simulink model "model1"  (R2019a)
settings: Solver=ode4  StartTime=0.0  StopTime=10.0  FixedStep=1E-3  RelTol=1e-3
values from neighbouring files (symbols this model uses):
  Kd = [3.0237 2.7708 7.5699 12.4043 5.742]    [code.m]    (also in matlab.mat)
  Ki = [1.5240 2.9039 1.9780 1.6885 2.8586]    [code.m]    (also in matlab.mat = [1.524 2.9039 1.978 1.6885 2.8586])
  Kp = [128.5204 102.3185 111.2328 109.4094 98.049]    [code.m]    (also in matlab.mat)
  Sce = Kd./(Kp*e_max)    [code.m]    (also in matlab.mat = [0.00235270042733 0.00270801467965 0.00680545666386 0.011337)
  Se = 1/e_max    (= 0.1)    [code.m]    (also in matlab.mat)
  Sie = Ki./(Kp*e_max)    [code.m]    (also in matlab.mat = [0.00118580396575 0.00283809868206 0.00177825245791 0.001543)
  Sout = e_max.*Kp    [code.m]    (also in matlab.mat = [1285.204 1023.185 1112.328 1094.094 980.49])
libraries: Fuzzy_Type2_Lib x5, simulink x5
settings Model: Creator=LENOVO  LastModifiedBy=LENOVO
settings DebuggingCC: UnderSpecifiedDimensionMsg=warning

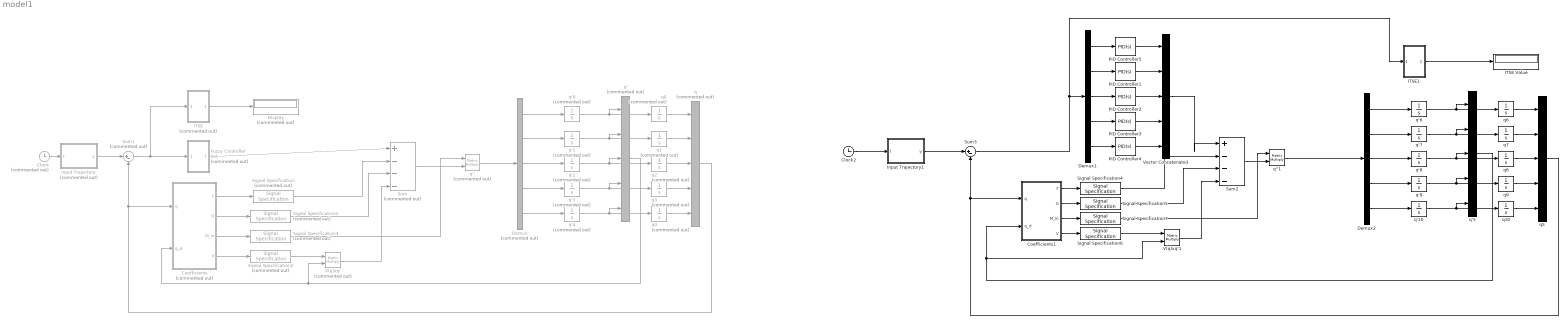
== system model1 ==
  Clock : Clock  Commented=on
  Clock2 : Clock
  Coefficients : MATLAB Function  Commented=on  TreatAsAtomicUnit=on
  Coefficients1 : MATLAB Function  TreatAsAtomicUnit=on
  Demux : Demux  Commented=on  Outputs=5
  Demux1 : Demux  Outputs=5
  Demux2 : Demux  Outputs=5
  Display : Display  Commented=on
  Fuzzy Controller Set : Subsystem  Commented=on
  ITSE : Subsystem  Commented=on
  ITSE Value : Display
  ITSE1 : Subsystem
  Input Trajectory : MATLAB Function  Commented=on  TreatAsAtomicUnit=on
  Input Trajectory1 : MATLAB Function  TreatAsAtomicUnit=on
  PID Controller1 : simulink/Continuous/PID Controller  Controller=PID  Form=Parallel  TimeDomain=Continuous-time  SampleTime=-1  IntegratorMethod=Forward Euler  FilterMethod=Forward Euler  ControllerParametersSource=internal  P=Kp(2)  I=Ki(2)  D=Kd(2)  UseFilter=on  N=100  TunerSelectOption=Transfer Function Based (PID Tuner App)  InitialConditionSource=internal  InitialConditionForIntegrator=0  InitialConditionForFilter=0  DifferentiatorICPrevScaledInput=0  ExternalReset=none  TrackingMode=off  Kt=1  LimitOutput=off  UpperSaturationLimit=inf  LowerSaturationLimit=-inf  LinearizeAsGain=on  AntiWindupMode=none  Kb=1  POutMin=[]  POutMax=[]  IOutMin=[]  IOutMax=[]  DOutMin=[]  DOutMax=[]  NOutMin=[]  NOutMax=[]  SumOutMin=[]  SumOutMax=[]  SaturationOutMin=[]  SaturationOutMax=[]  PParamMin=[]  PParamMax=[]  IParamMin=[]  IParamMax=[]  DParamMin=[]  DParamMax=[]  NParamMin=[]  NParamMax=[]  KbParamMin=[]  KbParamMax=[]  KtParamMin=[]  KtParamMax=[]  KbOutMin=[]  KbOutMax=[]  KtOutMin=[]  KtOutMax=[]  IntegratorOutMin=[]  IntegratorOutMax=[]  FilterOutMin=[]  FilterOutMax=[]  SumI1OutMin=[]  SumI1OutMax=[]  SumI2OutMin=[]  SumI2OutMax=[]  SumI3OutMin=[]  SumI3OutMax=[]  SumI4OutMin=[]  SumI4OutMax=[]  SumDOutMin=[]  SumDOutMax=[]  DifferentiatorOutMin=[]  DifferentiatorOutMax=[]  FilterDiffOutCoefMin=[]  FilterDiffOutCoefMax=[]  ReciprocalOutMin=[]  ReciprocalOutMax=[]  SumDenOutMin=[]  SumDenOutMax=[]  SumNumOutMin=[]  SumNumOutMax=[]  DivideOutMin=[]  DivideOutMax=[]  IntegratorContinuousStateAttributes=''  IntegratorStateMustResolveToSignalObject=off  IntegratorRTWStateStorageClass=Auto  FilterContinuousStateAttributes=''  FilterStateMustResolveToSignalObject=off  FilterRTWStateStorageClass=Auto  ParallelPVariant=InternalParameters  IdealPVariant=Disabled  IVariant=InternalParameters  DVariant=InternalParameters  IntegratorVariant=Continuous  SatVariant=Disabled  AWVariant=Passthrough  PCopyVariant=Disabled  TRVariant=Disabled  FdbkBlocksVariant=Forward  IdealPFdbkVariant=Disabled  SatFdbkVariant=Disabled  DerivativeFilterVariant=ContFilter  NVariant=InternalParameters  NCopyVariant=Disabled  FilterICVariant=InternalICsFilter  IntegratorICVariant=InternalICs  ExternalResetVariant=Disabled  TRSumVariant=Passthrough  SumFdbkVariant=Disabled  SumVariant=Sum_PID
  PID Controller2 : simulink/Continuous/PID Controller  Controller=PID  Form=Parallel  TimeDomain=Continuous-time  SampleTime=-1  IntegratorMethod=Forward Euler  FilterMethod=Forward Euler  ControllerParametersSource=internal  P=Kp(3)  I=Ki(3)  D=Kd(3)  UseFilter=on  N=100  TunerSelectOption=Transfer Function Based (PID Tuner App)  InitialConditionSource=internal  InitialConditionForIntegrator=0  InitialConditionForFilter=0  DifferentiatorICPrevScaledInput=0  ExternalReset=none  TrackingMode=off  Kt=1  LimitOutput=off  UpperSaturationLimit=inf  LowerSaturationLimit=-inf  LinearizeAsGain=on  AntiWindupMode=none  Kb=1  POutMin=[]  POutMax=[]  IOutMin=[]  IOutMax=[]  DOutMin=[]  DOutMax=[]  NOutMin=[]  NOutMax=[]  SumOutMin=[]  SumOutMax=[]  SaturationOutMin=[]  SaturationOutMax=[]  PParamMin=[]  PParamMax=[]  IParamMin=[]  IParamMax=[]  DParamMin=[]  DParamMax=[]  NParamMin=[]  NParamMax=[]  KbParamMin=[]  KbParamMax=[]  KtParamMin=[]  KtParamMax=[]  KbOutMin=[]  KbOutMax=[]  KtOutMin=[]  KtOutMax=[]  IntegratorOutMin=[]  IntegratorOutMax=[]  FilterOutMin=[]  FilterOutMax=[]  SumI1OutMin=[]  SumI1OutMax=[]  SumI2OutMin=[]  SumI2OutMax=[]  SumI3OutMin=[]  SumI3OutMax=[]  SumI4OutMin=[]  SumI4OutMax=[]  SumDOutMin=[]  SumDOutMax=[]  DifferentiatorOutMin=[]  DifferentiatorOutMax=[]  FilterDiffOutCoefMin=[]  FilterDiffOutCoefMax=[]  ReciprocalOutMin=[]  ReciprocalOutMax=[]  SumDenOutMin=[]  SumDenOutMax=[]  SumNumOutMin=[]  SumNumOutMax=[]  DivideOutMin=[]  DivideOutMax=[]  IntegratorContinuousStateAttributes=''  IntegratorStateMustResolveToSignalObject=off  IntegratorRTWStateStorageClass=Auto  FilterContinuousStateAttributes=''  FilterStateMustResolveToSignalObject=off  FilterRTWStateStorageClass=Auto  ParallelPVariant=InternalParameters  IdealPVariant=Disabled  IVariant=InternalParameters  DVariant=InternalParameters  IntegratorVariant=Continuous  SatVariant=Disabled  AWVariant=Passthrough  PCopyVariant=Disabled  TRVariant=Disabled  FdbkBlocksVariant=Forward  IdealPFdbkVariant=Disabled  SatFdbkVariant=Disabled  DerivativeFilterVariant=ContFilter  NVariant=InternalParameters  NCopyVariant=Disabled  FilterICVariant=InternalICsFilter  IntegratorICVariant=InternalICs  ExternalResetVariant=Disabled  TRSumVariant=Passthrough  SumFdbkVariant=Disabled  SumVariant=Sum_PID
  PID Controller3 : simulink/Continuous/PID Controller  Controller=PID  Form=Parallel  TimeDomain=Continuous-time  SampleTime=-1  IntegratorMethod=Forward Euler  FilterMethod=Forward Euler  ControllerParametersSource=internal  P=Kp(4)  I=Ki(4)  D=Kd(4)  UseFilter=on  N=100  TunerSelectOption=Transfer Function Based (PID Tuner App)  InitialConditionSource=internal  InitialConditionForIntegrator=0  InitialConditionForFilter=0  DifferentiatorICPrevScaledInput=0  ExternalReset=none  TrackingMode=off  Kt=1  LimitOutput=off  UpperSaturationLimit=inf  LowerSaturationLimit=-inf  LinearizeAsGain=on  AntiWindupMode=none  Kb=1  POutMin=[]  POutMax=[]  IOutMin=[]  IOutMax=[]  DOutMin=[]  DOutMax=[]  NOutMin=[]  NOutMax=[]  SumOutMin=[]  SumOutMax=[]  SaturationOutMin=[]  SaturationOutMax=[]  PParamMin=[]  PParamMax=[]  IParamMin=[]  IParamMax=[]  DParamMin=[]  DParamMax=[]  NParamMin=[]  NParamMax=[]  KbParamMin=[]  KbParamMax=[]  KtParamMin=[]  KtParamMax=[]  KbOutMin=[]  KbOutMax=[]  KtOutMin=[]  KtOutMax=[]  IntegratorOutMin=[]  IntegratorOutMax=[]  FilterOutMin=[]  FilterOutMax=[]  SumI1OutMin=[]  SumI1OutMax=[]  SumI2OutMin=[]  SumI2OutMax=[]  SumI3OutMin=[]  SumI3OutMax=[]  SumI4OutMin=[]  SumI4OutMax=[]  SumDOutMin=[]  SumDOutMax=[]  DifferentiatorOutMin=[]  DifferentiatorOutMax=[]  FilterDiffOutCoefMin=[]  FilterDiffOutCoefMax=[]  ReciprocalOutMin=[]  ReciprocalOutMax=[]  SumDenOutMin=[]  SumDenOutMax=[]  SumNumOutMin=[]  SumNumOutMax=[]  DivideOutMin=[]  DivideOutMax=[]  IntegratorContinuousStateAttributes=''  IntegratorStateMustResolveToSignalObject=off  IntegratorRTWStateStorageClass=Auto  FilterContinuousStateAttributes=''  FilterStateMustResolveToSignalObject=off  FilterRTWStateStorageClass=Auto  ParallelPVariant=InternalParameters  IdealPVariant=Disabled  IVariant=InternalParameters  DVariant=InternalParameters  IntegratorVariant=Continuous  SatVariant=Disabled  AWVariant=Passthrough  PCopyVariant=Disabled  TRVariant=Disabled  FdbkBlocksVariant=Forward  IdealPFdbkVariant=Disabled  SatFdbkVariant=Disabled  DerivativeFilterVariant=ContFilter  NVariant=InternalParameters  NCopyVariant=Disabled  FilterICVariant=InternalICsFilter  IntegratorICVariant=InternalICs  ExternalResetVariant=Disabled  TRSumVariant=Passthrough  SumFdbkVariant=Disabled  SumVariant=Sum_PID
  PID Controller4 : simulink/Continuous/PID Controller  Controller=PID  Form=Parallel  TimeDomain=Continuous-time  SampleTime=-1  IntegratorMethod=Forward Euler  FilterMethod=Forward Euler  ControllerParametersSource=internal  P=Kp(5)  I=Ki(5)  D=Kd(5)  UseFilter=on  N=100  TunerSelectOption=Transfer Function Based (PID Tuner App)  InitialConditionSource=internal  InitialConditionForIntegrator=0  InitialConditionForFilter=0  DifferentiatorICPrevScaledInput=0  ExternalReset=none  TrackingMode=off  Kt=1  LimitOutput=off  UpperSaturationLimit=inf  LowerSaturationLimit=-inf  LinearizeAsGain=on  AntiWindupMode=none  Kb=1  POutMin=[]  POutMax=[]  IOutMin=[]  IOutMax=[]  DOutMin=[]  DOutMax=[]  NOutMin=[]  NOutMax=[]  SumOutMin=[]  SumOutMax=[]  SaturationOutMin=[]  SaturationOutMax=[]  PParamMin=[]  PParamMax=[]  IParamMin=[]  IParamMax=[]  DParamMin=[]  DParamMax=[]  NParamMin=[]  NParamMax=[]  KbParamMin=[]  KbParamMax=[]  KtParamMin=[]  KtParamMax=[]  KbOutMin=[]  KbOutMax=[]  KtOutMin=[]  KtOutMax=[]  IntegratorOutMin=[]  IntegratorOutMax=[]  FilterOutMin=[]  FilterOutMax=[]  SumI1OutMin=[]  SumI1OutMax=[]  SumI2OutMin=[]  SumI2OutMax=[]  SumI3OutMin=[]  SumI3OutMax=[]  SumI4OutMin=[]  SumI4OutMax=[]  SumDOutMin=[]  SumDOutMax=[]  DifferentiatorOutMin=[]  DifferentiatorOutMax=[]  FilterDiffOutCoefMin=[]  FilterDiffOutCoefMax=[]  ReciprocalOutMin=[]  ReciprocalOutMax=[]  SumDenOutMin=[]  SumDenOutMax=[]  SumNumOutMin=[]  SumNumOutMax=[]  DivideOutMin=[]  DivideOutMax=[]  IntegratorContinuousStateAttributes=''  IntegratorStateMustResolveToSignalObject=off  IntegratorRTWStateStorageClass=Auto  FilterContinuousStateAttributes=''  FilterStateMustResolveToSignalObject=off  FilterRTWStateStorageClass=Auto  ParallelPVariant=InternalParameters  IdealPVariant=Disabled  IVariant=InternalParameters  DVariant=InternalParameters  IntegratorVariant=Continuous  SatVariant=Disabled  AWVariant=Passthrough  PCopyVariant=Disabled  TRVariant=Disabled  FdbkBlocksVariant=Forward  IdealPFdbkVariant=Disabled  SatFdbkVariant=Disabled  DerivativeFilterVariant=ContFilter  NVariant=InternalParameters  NCopyVariant=Disabled  FilterICVariant=InternalICsFilter  IntegratorICVariant=InternalICs  ExternalResetVariant=Disabled  TRSumVariant=Passthrough  SumFdbkVariant=Disabled  SumVariant=Sum_PID
  PID Controller5 : simulink/Continuous/PID Controller  Controller=PID  Form=Parallel  TimeDomain=Continuous-time  SampleTime=-1  IntegratorMethod=Forward Euler  FilterMethod=Forward Euler  ControllerParametersSource=internal  P=Kp(1)  I=Ki(1)  D=Kd(1)  UseFilter=on  N=100  TunerSelectOption=Transfer Function Based (PID Tuner App)  InitialConditionSource=internal  InitialConditionForIntegrator=0  InitialConditionForFilter=0  DifferentiatorICPrevScaledInput=0  ExternalReset=none  TrackingMode=off  Kt=1  LimitOutput=off  UpperSaturationLimit=inf  LowerSaturationLimit=-inf  LinearizeAsGain=on  AntiWindupMode=none  Kb=1  POutMin=[]  POutMax=[]  IOutMin=[]  IOutMax=[]  DOutMin=[]  DOutMax=[]  NOutMin=[]  NOutMax=[]  SumOutMin=[]  SumOutMax=[]  SaturationOutMin=[]  SaturationOutMax=[]  PParamMin=[]  PParamMax=[]  IParamMin=[]  IParamMax=[]  DParamMin=[]  DParamMax=[]  NParamMin=[]  NParamMax=[]  KbParamMin=[]  KbParamMax=[]  KtParamMin=[]  KtParamMax=[]  KbOutMin=[]  KbOutMax=[]  KtOutMin=[]  KtOutMax=[]  IntegratorOutMin=[]  IntegratorOutMax=[]  FilterOutMin=[]  FilterOutMax=[]  SumI1OutMin=[]  SumI1OutMax=[]  SumI2OutMin=[]  SumI2OutMax=[]  SumI3OutMin=[]  SumI3OutMax=[]  SumI4OutMin=[]  SumI4OutMax=[]  SumDOutMin=[]  SumDOutMax=[]  DifferentiatorOutMin=[]  DifferentiatorOutMax=[]  FilterDiffOutCoefMin=[]  FilterDiffOutCoefMax=[]  ReciprocalOutMin=[]  ReciprocalOutMax=[]  SumDenOutMin=[]  SumDenOutMax=[]  SumNumOutMin=[]  SumNumOutMax=[]  DivideOutMin=[]  DivideOutMax=[]  IntegratorContinuousStateAttributes=''  IntegratorStateMustResolveToSignalObject=off  IntegratorRTWStateStorageClass=Auto  FilterContinuousStateAttributes=''  FilterStateMustResolveToSignalObject=off  FilterRTWStateStorageClass=Auto  ParallelPVariant=InternalParameters  IdealPVariant=Disabled  IVariant=InternalParameters  DVariant=InternalParameters  IntegratorVariant=Continuous  SatVariant=Disabled  AWVariant=Passthrough  PCopyVariant=Disabled  TRVariant=Disabled  FdbkBlocksVariant=Forward  IdealPFdbkVariant=Disabled  SatFdbkVariant=Disabled  DerivativeFilterVariant=ContFilter  NVariant=InternalParameters  NCopyVariant=Disabled  FilterICVariant=InternalICsFilter  IntegratorICVariant=InternalICs  ExternalResetVariant=Disabled  TRSumVariant=Passthrough  SumFdbkVariant=Disabled  SumVariant=Sum_PID
  Signal Specification : SignalSpecification  Commented=on  Dimensions=[5 1]
  Signal Specification1 : SignalSpecification  Commented=on  Dimensions=[5 1]
  Signal Specification2 : SignalSpecification  Commented=on  Dimensions=[5 5]
  Signal Specification3 : SignalSpecification  Commented=on  Dimensions=[5 5]
  Signal Specification4 : SignalSpecification  Dimensions=[5 1]
  Signal Specification5 : SignalSpecification  Dimensions=[5 1]
  Signal Specification6 : SignalSpecification  Dimensions=[5 5]
  Signal Specification7 : SignalSpecification  Dimensions=[5 5]
  Sum : Sum  Commented=on  Inputs=|+---
  Sum1 : Sum  Commented=on  Inputs=|+-  InputSameDT=on
  Sum2 : Sum  Inputs=|+---
  Sum3 : Sum  Inputs=|+-  InputSameDT=on
  V(q)xq' : Product  Commented=on  Multiplication=Matrix(*)
  V(q)xq'1 : Product  Multiplication=Matrix(*)
  Vector Concatenate3 : Concatenate  NumInputs=5  Mode=Multidimensional array
  q : Concatenate  Commented=on  NumInputs=5  Mode=Multidimensional array
  q' : Concatenate  Commented=on  NumInputs=5  Mode=Multidimensional array
  q'' : Product  Commented=on  Multiplication=Matrix(*)
  q''1 : Product  Multiplication=Matrix(*)
  q'{0..4} (5 alike) : Integrator  Commented=on
  q'{6..10} (5 alike) : Integrator
  q'5 : Concatenate  NumInputs=5  Mode=Multidimensional array
  q{0..4} (5 alike) : Integrator  Commented=on
  q{6..10} (5 alike) : Integrator
  q5 : Concatenate  NumInputs=5  Mode=Multidimensional array
  wires:
  Coefficients/1(F) -> Signal Specification/1
  Coefficients/2(G) -> Signal Specification1/1
  q'0/1 -> q'/1, q0/1
  V(q)xq'/1 -> Sum/4
  q''/1 -> Demux/1
  Coefficients/3(M_in) -> Signal Specification3/1
  Sum/1 -> q''/2
  q2/1 -> q/3
  Input Trajectory/1(y) -> Sum1/1
  q'3/1 -> q'/4, q3/1
  q'4/1 -> q'/5, q4/1
  q'2/1 -> q'/3, q2/1
  q'1/1 -> q'/2, q1/1
  q'/1 -> Coefficients/2(q_d), V(q)xq'/2
  q0/1 -> q/1
  q1/1 -> q/2
  q3/1 -> q/4
  q4/1 -> q/5
  q/1 -> Sum1/2, Coefficients/1(q)
  Demux/1 -> q'0/1
  Demux/2 -> q'1/1
  Demux/3 -> q'2/1
  Demux/4 -> q'3/1
  Demux/5 -> q'4/1
  Sum1/1 -> Fuzzy Controller Set/1(Input), ITSE/1(Input)
  ITSE/1(Output) -> Display/1
  ITSE1/1(Output) -> ITSE Value/1
  Demux2/5 -> q'10/1
  Demux2/4 -> q'9/1
  Demux2/3 -> q'8/1
  Demux2/2 -> q'7/1
  Demux2/1 -> q'6/1
  q5/1 -> Sum3/2, Coefficients1/1(q)
  q10/1 -> q5/5
  q9/1 -> q5/4
  q7/1 -> q5/2
  q6/1 -> q5/1
  q'5/1 -> V(q)xq'1/2, Coefficients1/2(q_d)
  q'7/1 -> q7/1, q'5/2
  q'8/1 -> q8/1, q'5/3
  q'10/1 -> q10/1, q'5/5
  q'9/1 -> q9/1, q'5/4
  Clock2/1 -> Input Trajectory1/1(t)
  Input Trajectory1/1(y) -> Sum3/1
  q8/1 -> q5/3
  Sum2/1 -> q''1/2
  Coefficients1/3(M_in) -> Signal Specification7/1
  q''1/1 -> Demux2/1
  V(q)xq'1/1 -> Sum2/4
  q'6/1 -> q6/1, q'5/1
  Coefficients1/2(G) -> Signal Specification5/1
  Coefficients1/1(F) -> Signal Specification4/1
  Signal Specification/1 -> Sum/2
  Signal Specification1/1 -> Sum/3
  Signal Specification3/1 -> q''/1
  Coefficients/4(V) -> Signal Specification2/1
  Signal Specification2/1 -> V(q)xq'/1
  Signal Specification4/1 -> Sum2/2
  Signal Specification5/1 -> Sum2/3
  Signal Specification7/1 -> q''1/1
  Signal Specification6/1 -> V(q)xq'1/1
  Coefficients1/4(V) -> Signal Specification6/1
  Sum3/1 -> Demux1/1, ITSE1/1(Input)
  PID Controller1/1 -> Vector Concatenate3/2
  Vector Concatenate3/1 -> Sum2/1
  Demux1/2 -> PID Controller1/1
  PID Controller3/1 -> Vector Concatenate3/4
  PID Controller4/1 -> Vector Concatenate3/5
  Demux1/4 -> PID Controller3/1
  PID Controller5/1 -> Vector Concatenate3/1
  Demux1/1 -> PID Controller5/1
  Demux1/5 -> PID Controller4/1
  PID Controller2/1 -> Vector Concatenate3/3
  Demux1/3 -> PID Controller2/1
  Fuzzy Controller Set/1(Output) -> Sum/1
  Clock/1 -> Input Trajectory/1(t)

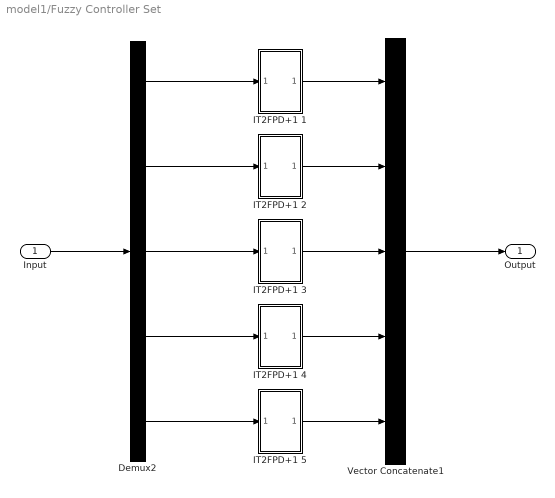
== system model1/Fuzzy Controller Set ==
  Input : Inport
  Demux2 : Demux  Outputs=5
  IT2FPD+1 1 : Subsystem
  IT2FPD+1 2 : Subsystem
  IT2FPD+1 3 : Subsystem
  IT2FPD+1 4 : Subsystem
  IT2FPD+1 5 : Subsystem
  Vector Concatenate1 : Concatenate  NumInputs=5  Mode=Multidimensional array
  Output : Outport
  wires:
  Demux2/3 -> IT2FPD+1 3/1(Input)
  Demux2/5 -> IT2FPD+1 5/1(Input)
  Demux2/2 -> IT2FPD+1 2/1(Input)
  Demux2/4 -> IT2FPD+1 4/1(Input)
  IT2FPD+1 4/1(Output) -> Vector Concatenate1/4
  Input/1 -> Demux2/1
  Vector Concatenate1/1 -> Output/1
  Demux2/1 -> IT2FPD+1 1/1(Input)
  IT2FPD+1 2/1(Output) -> Vector Concatenate1/2
  IT2FPD+1 1/1(Output) -> Vector Concatenate1/1
  IT2FPD+1 3/1(Output) -> Vector Concatenate1/3
  IT2FPD+1 5/1(Output) -> Vector Concatenate1/5

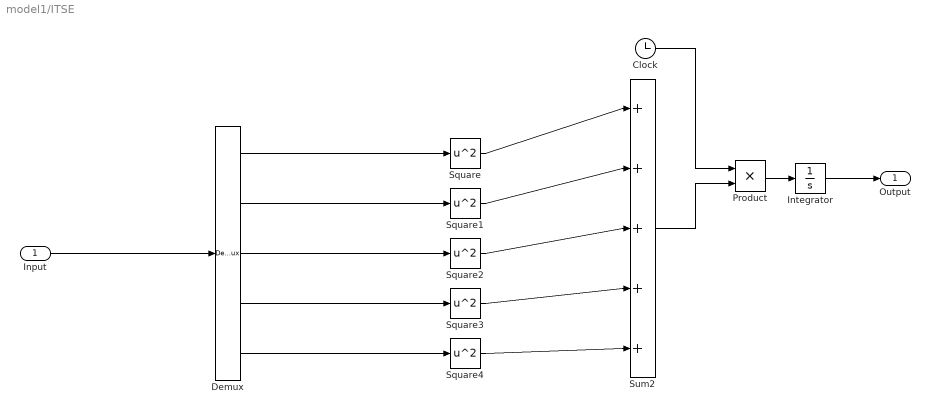
== system model1/ITSE ==
  Input : Inport
  Clock : Clock
  Demux : Demux  Outputs=5
  Integrator : Integrator
  Product : Product
  Square{,1..4} (5 alike) : Math  Operator=square  SaturateOnIntegerOverflow=on
  Sum2 : Sum  Inputs=|+++++
  Output : Outport
  wires:
  Sum2/1 -> Product/2
  Integrator/1 -> Output/1
  Product/1 -> Integrator/1
  Square1/1 -> Sum2/2
  Square/1 -> Sum2/1
  Square2/1 -> Sum2/3
  Square4/1 -> Sum2/5
  Square3/1 -> Sum2/4
  Demux/1 -> Square/1
  Demux/2 -> Square1/1
  Demux/3 -> Square2/1
  Demux/4 -> Square3/1
  Demux/5 -> Square4/1
  Clock/1 -> Product/1
  Input/1 -> Demux/1

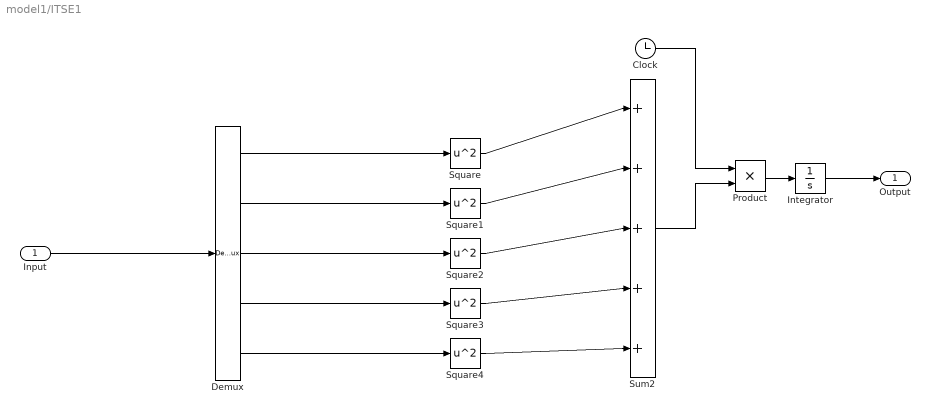
== system model1/ITSE1 ==
  Input : Inport
  Clock : Clock
  Demux : Demux  Outputs=5
  Integrator : Integrator
  Product : Product
  Square{,1..4} (5 alike) : Math  Operator=square  SaturateOnIntegerOverflow=on
  Sum2 : Sum  Inputs=|+++++
  Output : Outport
  wires:
  Input/1 -> Demux/1
  Clock/1 -> Product/1
  Demux/5 -> Square4/1
  Demux/4 -> Square3/1
  Demux/3 -> Square2/1
  Demux/2 -> Square1/1
  Demux/1 -> Square/1
  Square3/1 -> Sum2/4
  Square4/1 -> Sum2/5
  Square2/1 -> Sum2/3
  Square/1 -> Sum2/1
  Square1/1 -> Sum2/2
  Product/1 -> Integrator/1
  Integrator/1 -> Output/1
  Sum2/1 -> Product/2

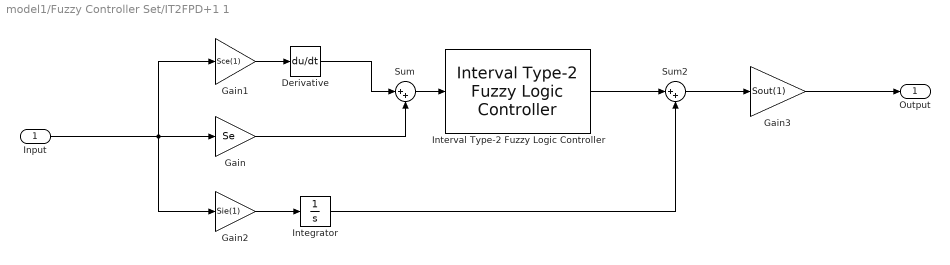
== system model1/Fuzzy Controller Set/IT2FPD+1 1 ==
  Input : Inport
  Derivative : Derivative
  Gain : Gain  Gain=Se
  Gain1 : Gain  Gain=Sce(1)
  Gain2 : Gain  Gain=Sie(1)
  Gain3 : Gain  Gain=Sout(1)
  Integrator : Integrator
  Interval Type-2 Fuzzy Logic Controller : Fuzzy_Type2_Lib/Interval Type-2 Fuzzy Logic Controller  t2fisSim=Fuzzy_PD.fis
      settings: SourceProductName=Interval Type-2 Fuzzy Logic Systems Toolbox
  Sum : Sum  Inputs=|++
  Sum2 : Sum  Inputs=|++
  Output : Outport
  wires:
  Derivative/1 -> Sum/1
  Gain3/1 -> Output/1
  Sum2/1 -> Gain3/1
  Input/1 -> Gain2/1, Gain/1, Gain1/1
  Gain1/1 -> Derivative/1
  Interval Type-2 Fuzzy Logic Controller/1 -> Sum2/1
  Gain/1 -> Sum/2
  Gain2/1 -> Integrator/1
  Integrator/1 -> Sum2/2
  Sum/1 -> Interval Type-2 Fuzzy Logic Controller/1

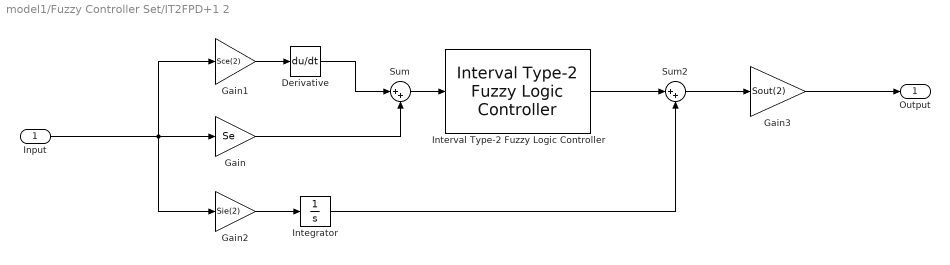
== system model1/Fuzzy Controller Set/IT2FPD+1 2 ==
  Input : Inport
  Derivative : Derivative
  Gain : Gain  Gain=Se
  Gain1 : Gain  Gain=Sce(2)
  Gain2 : Gain  Gain=Sie(2)
  Gain3 : Gain  Gain=Sout(2)
  Integrator : Integrator
  Interval Type-2 Fuzzy Logic Controller : Fuzzy_Type2_Lib/Interval Type-2 Fuzzy Logic Controller  t2fisSim=Fuzzy_PD.fis
      settings: SourceProductName=Interval Type-2 Fuzzy Logic Systems Toolbox
  Sum : Sum  Inputs=|++
  Sum2 : Sum  Inputs=|++
  Output : Outport
  wires:
  Integrator/1 -> Sum2/2
  Gain2/1 -> Integrator/1
  Interval Type-2 Fuzzy Logic Controller/1 -> Sum2/1
  Gain1/1 -> Derivative/1
  Input/1 -> Gain1/1, Gain/1, Gain2/1
  Sum2/1 -> Gain3/1
  Gain3/1 -> Output/1
  Derivative/1 -> Sum/1
  Gain/1 -> Sum/2
  Sum/1 -> Interval Type-2 Fuzzy Logic Controller/1

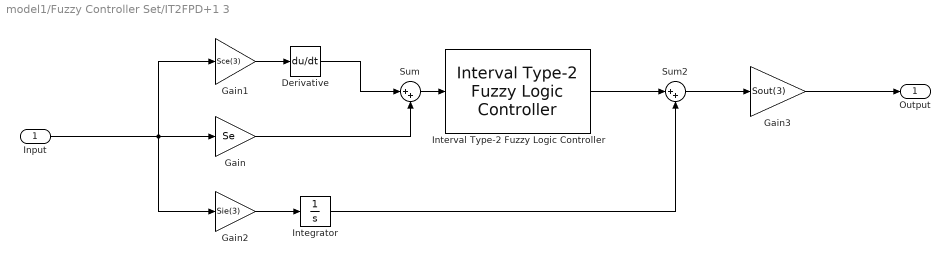
== system model1/Fuzzy Controller Set/IT2FPD+1 3 ==
  Input : Inport
  Derivative : Derivative
  Gain : Gain  Gain=Se
  Gain1 : Gain  Gain=Sce(3)
  Gain2 : Gain  Gain=Sie(3)
  Gain3 : Gain  Gain=Sout(3)
  Integrator : Integrator
  Interval Type-2 Fuzzy Logic Controller : Fuzzy_Type2_Lib/Interval Type-2 Fuzzy Logic Controller  t2fisSim=Fuzzy_PD.fis
      settings: SourceProductName=Interval Type-2 Fuzzy Logic Systems Toolbox
  Sum : Sum  Inputs=|++
  Sum2 : Sum  Inputs=|++
  Output : Outport
  wires:
  Derivative/1 -> Sum/1
  Gain3/1 -> Output/1
  Sum2/1 -> Gain3/1
  Input/1 -> Gain2/1, Gain/1, Gain1/1
  Gain1/1 -> Derivative/1
  Interval Type-2 Fuzzy Logic Controller/1 -> Sum2/1
  Gain2/1 -> Integrator/1
  Integrator/1 -> Sum2/2
  Gain/1 -> Sum/2
  Sum/1 -> Interval Type-2 Fuzzy Logic Controller/1

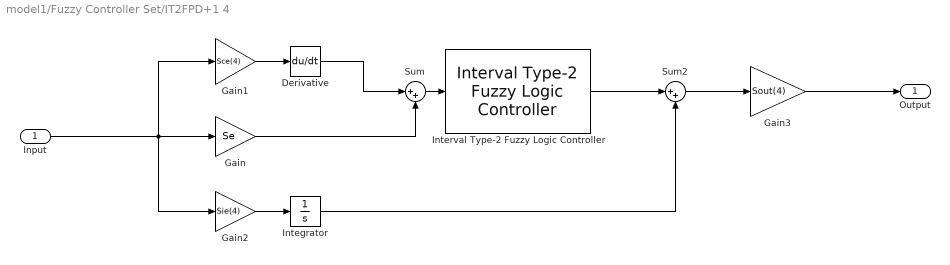
== system model1/Fuzzy Controller Set/IT2FPD+1 4 ==
  Input : Inport
  Derivative : Derivative
  Gain : Gain  Gain=Se
  Gain1 : Gain  Gain=Sce(4)
  Gain2 : Gain  Gain=Sie(4)
  Gain3 : Gain  Gain=Sout(4)
  Integrator : Integrator
  Interval Type-2 Fuzzy Logic Controller : Fuzzy_Type2_Lib/Interval Type-2 Fuzzy Logic Controller  t2fisSim=Fuzzy_PD.fis
      settings: SourceProductName=Interval Type-2 Fuzzy Logic Systems Toolbox
  Sum : Sum  Inputs=|++
  Sum2 : Sum  Inputs=|++
  Output : Outport
  wires:
  Integrator/1 -> Sum2/2
  Gain2/1 -> Integrator/1
  Interval Type-2 Fuzzy Logic Controller/1 -> Sum2/1
  Gain1/1 -> Derivative/1
  Input/1 -> Gain1/1, Gain/1, Gain2/1
  Sum2/1 -> Gain3/1
  Gain3/1 -> Output/1
  Derivative/1 -> Sum/1
  Gain/1 -> Sum/2
  Sum/1 -> Interval Type-2 Fuzzy Logic Controller/1

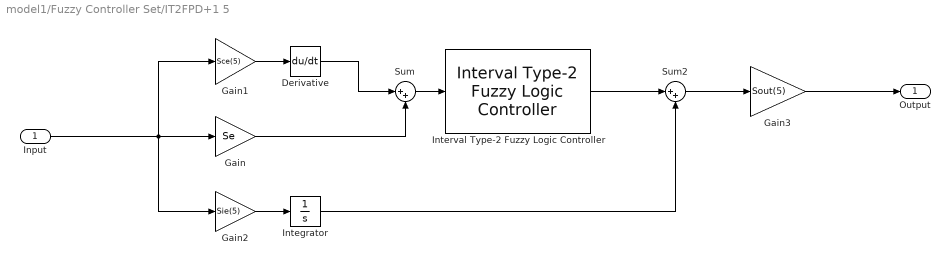
== system model1/Fuzzy Controller Set/IT2FPD+1 5 ==
  Input : Inport
  Derivative : Derivative
  Gain : Gain  Gain=Se
  Gain1 : Gain  Gain=Sce(5)
  Gain2 : Gain  Gain=Sie(5)
  Gain3 : Gain  Gain=Sout(5)
  Integrator : Integrator
  Interval Type-2 Fuzzy Logic Controller : Fuzzy_Type2_Lib/Interval Type-2 Fuzzy Logic Controller  t2fisSim=Fuzzy_PD.fis
      settings: SourceProductName=Interval Type-2 Fuzzy Logic Systems Toolbox
  Sum : Sum  Inputs=|++
  Sum2 : Sum  Inputs=|++
  Output : Outport
  wires:
  Derivative/1 -> Sum/1
  Gain3/1 -> Output/1
  Sum2/1 -> Gain3/1
  Input/1 -> Gain2/1, Gain/1, Gain1/1
  Gain1/1 -> Derivative/1
  Interval Type-2 Fuzzy Logic Controller/1 -> Sum2/1
  Gain2/1 -> Integrator/1
  Integrator/1 -> Sum2/2
  Gain/1 -> Sum/2
  Sum/1 -> Interval Type-2 Fuzzy Logic Controller/1

== matlab function model1/Coefficients ==
  data: F output; G output; q input; M_in output; q_d input; V output
function [F, G, M_in, V] = fcn(q, q_d)

%%%%%%%%%%%%%%%%%%%%%%%%%%%%%%%%%%%%%%%%%%%%
%% Defining SCARA 5-DOF manipulator parameters 

l = [ 0.524, 0.2, 0.2, 0.2, 0.14];
lc= [0 , 0.0229, 0.0229, 0.0229, 0];
m = [1.228, 1.023, 1.023, 1.023, 0.5114];
Izz = [0, 0.0058, 0.0058, 0.0058, 0];
Fv = [0.03, 0.025, 0.025, 0.025, 0.02];

link_parameters = [l ; lc; m ; Izz; Fv];

%%
M= zeros(5,5);
%Populating inertia (M) matrix
M(1,1) = sum(m);
M(1,5) = -m(5);
M(5,1) = -m(5);
M(5,5)= m(5);
M(4,4) = (lc(4)^2)*m(4) + (l(4)^2)*m(5) + Izz(4);
M(3,4) = ((lc(4)^2)+ (l(3)*lc(4)*cos(q(4))))*m(4)+ ((l(4)^2)+(l(3)*l(4)*cos(q(4))))*m(5) + Izz(4);
M(4,3)= M(3,4);
M(2,3)= ((lc(3)^2)+(l(2)*lc(3)*cos(q(3))))*m(3) + ((l(3)^2)+(lc(4)^2)+(l(2)*l(3)*cos(q(3)))+(2*l(3)*lc(4)*cos(q(4)))+(l(2)*lc(4)*cos(q(3)+q(4))))*m(4) + ((l(2)*l(4)*cos(q(3)+q(4)))+(l(3)^2)+(l(4)^2)+(l(2)*l(3)*cos(q(3)))+(2*l(3)*l(4)*cos(q(4))))*m(5) + Izz(3) + Izz(4); 
M(3,2) = M(2,3);
M(2,2) =  ((lc(2)^2))*m(2) + ((l(2)^2)+(lc(3)^2)+ (2*l(2)*lc(3)*cos(q(3))))*m(3) + ((l(2)^2)+(l(3)^2)+(lc(4)^2)+(2*l(2)*l(3)*cos(q(3))) + (2*l(3)*lc(4)*cos(q(4))) + (2*l(2)*lc(4)*cos(q(3)+q(4))))*m(4) +  ((l(2)^2)+(l(3)^2)+(l(4)^2)+(2*l(2)*l(3)*cos(q(3))) + (2*l(3)*l(4)*cos(q(4))) + (2*l(2)*l(4)*cos(q(3)+q(4))))*m(5) + Izz(2) + Izz(3) + Izz(4);
M(3,3)= ((lc(3)^2))*m(3) + ((l(3)^2)+(lc(4)^2)+(2*l(3)*lc(4)*cos(q(4))))*m(4) + ((l(3)^2)+(lc(4)^2)+(2*l(4)*lc(4)))*m(5) + Izz(3) + Izz(4);
M(4,2) = ((lc(4)^2)+(l(3)*lc(4)*cos(q(4)))+(l(2)*lc(4)*cos(q(3)+q(4))))*m(4) + ((l(4)^2)+(l(3)*l(4)*cos(q(4)))+(l(2)*l(4)*cos(q(3)+q(4))))*m(5)+Izz(4);
M(2,4)=M(4,2);


M_in = inv(M);

%% 
V= zeros(5,5);
%Populating V matrix
V(2,2) = -((lc(3)*m(3))+ (l(3)*m(4)) + (l(3)*m(5)))*l(2)*sin(q(3))*q_d(3) + ((l(2)*sin(q(3)+q(4))*(q_d(3)-q_d(4)))-((l(3)*sin(q(4))*q_d(4))))*(lc(4)*m(4)+l(4)*m(5));
V(2,3) = -((lc(3)*m(3))+(l(3)*m(4))+(l(3)*m(5)))*(l(2)*sin(q(3))*q_d(2)) -((lc(4)*m(4))+(l(4)*m(5)))*(l(2)*sin(q(3)+q(4))*q_d(2))-((lc(3)*m(3))+(l(3)*m(4))+(l(3)*m(5)))*(l(2)*sin(q(3))*q_d(3)) - ((lc(4)*m(4))+(l(4)*m(5)))*(l(2)*sin(q(3)+q(4))*q_d(3))-((lc(4)*m(4))+(l(4)*m(5)))*((l(3)*sin(q(4)))+(l(2)*sin(q(3)+q(4)))*q_d(4));
V(2,4) = -((lc(4)*m(4))+(l(4)*m(5)))*((l(3)*sin(q(4)))+(l(2)*sin(q(3)+q(4))))*(q_d(3)+q_d(4)+q_d(2));
V(3,2) = ((lc(3)*m(3))+(l(3)*m(4))+(l(3)*m(5)))*(l(2)*sin(q(3))*q_d(2)) + ((lc(4)*m(4))+(l(4)*m(5)))*(l(2)*sin(q(3)+q(4))*q_d(2))-((lc(4)*m(4))+(l(4)*m(5)))*l(3)*sin(q(4))*q_d(4);
V(3,3) = -((lc(4)*m(4))+l(4)*m(5))*l(3)*sin(q(4))*q_d(4);
V(3,4) = -((lc(4)*m(4))+l(4)*m(5))*l(3)*sin(q(4))*(q_d(2)+q_d(3)+q_d(4));
V(4,2) = ((lc(4)*m(4))+l(4)*m(5))*((((l(2)*sin(q(3)+q(4)))+(l(3)*sin(q(4))))*q_d(2)) + (l(3)*sin(q(4))*q_d(3)));
V(4,3) =  ((lc(4)*m(4))+l(4)*m(5))*l(3)*sin(q(4))*(q_d(2)+q_d(3));

%%
gz= 9.8;
G = zeros(5,1);
%Populating gravitational force (G) matrix
G = [sum(m)*gz; 0; 0; 0; -m(5)*gz];

%%

F = zeros(5,1);
%Populating Friction (F) matrix
F = [(Fv(1)*q_d(1)); (Fv(2)*q_d(2)); (Fv(3)*q_d(3)); (Fv(4)*q_d(4)); (Fv(5)*q_d(5))];

end

== matlab function model1/Coefficients1 ==
  data: F output; G output; q input; M_in output; q_d input; V output
function [F, G, M_in, V] = fcn(q, q_d)


%%%%%%%%%%%%%%%%%%%%%%%%%%%%%%%%%%%%%%%%%%%%
%% Defining SCARA 5-DOF manipulator parameters 

l = [ 0.524, 0.2, 0.2, 0.2, 0.14];
lc= [0 , 0.0229, 0.0229, 0.0229, 0];
m = [1.228, 1.023, 1.023, 1.023, 0.5114];
Izz = [0, 0.0058, 0.0058, 0.0058, 0];
Fv = [0.03, 0.025, 0.025, 0.025, 0.02];

link_parameters = [l ; lc; m ; Izz; Fv];

%%
M= zeros(5,5);
%Populating inertia (M) matrix
M(1,1) = sum(m);
M(1,5) = -m(5);
M(5,1) = -m(5);
M(5,5)= m(5);
M(4,4) = (lc(4)^2)*m(4) + (l(4)^2)*m(5) + Izz(4);
M(3,4) = ((lc(4)^2)+ (l(3)*lc(4)*cos(q(4))))*m(4)+ ((l(4)^2)+(l(3)*l(4)*cos(q(4))))*m(5) + Izz(4);
M(4,3)= M(3,4);
M(2,3)= ((lc(3)^2)+(l(2)*lc(3)*cos(q(3))))*m(3) + ((l(3)^2)+(lc(4)^2)+(l(2)*l(3)*cos(q(3)))+(2*l(3)*lc(4)*cos(q(4)))+(l(2)*lc(4)*cos(q(3)+q(4))))*m(4) + ((l(2)*l(4)*cos(q(3)+q(4)))+(l(3)^2)+(l(4)^2)+(l(2)*l(3)*cos(q(3)))+(2*l(3)*l(4)*cos(q(4))))*m(5) + Izz(3) + Izz(4); 
M(3,2) = M(2,3);
M(2,2) =  ((lc(2)^2))*m(2) + ((l(2)^2)+(lc(3)^2)+ (2*l(2)*lc(3)*cos(q(3))))*m(3) + ((l(2)^2)+(l(3)^2)+(lc(4)^2)+(2*l(2)*l(3)*cos(q(3))) + (2*l(3)*lc(4)*cos(q(4))) + (2*l(2)*lc(4)*cos(q(3)+q(4))))*m(4) +  ((l(2)^2)+(l(3)^2)+(l(4)^2)+(2*l(2)*l(3)*cos(q(3))) + (2*l(3)*l(4)*cos(q(4))) + (2*l(2)*l(4)*cos(q(3)+q(4))))*m(5) + Izz(2) + Izz(3) + Izz(4);
M(3,3)= ((lc(3)^2))*m(3) + ((l(3)^2)+(lc(4)^2)+(2*l(3)*lc(4)*cos(q(4))))*m(4) + ((l(3)^2)+(lc(4)^2)+(2*l(4)*lc(4)))*m(5) + Izz(3) + Izz(4);
M(4,2) = ((lc(4)^2)+(l(3)*lc(4)*cos(q(4)))+(l(2)*lc(4)*cos(q(3)+q(4))))*m(4) + ((l(4)^2)+(l(3)*l(4)*cos(q(4)))+(l(2)*l(4)*cos(q(3)+q(4))))*m(5)+Izz(4);
M(2,4)=M(4,2);


M_in = inv(M);

%% 
V= zeros(5,5);
%Populating V matrix
V(2,2) = -((lc(3)*m(3))+ (l(3)*m(4)) + (l(3)*m(5)))*l(2)*sin(q(3))*q_d(3) + ((l(2)*sin(q(3)+q(4))*(q_d(3)-q_d(4)))-((l(3)*sin(q(4))*q_d(4))))*(lc(4)*m(4)+l(4)*m(5));
V(2,3) = -((lc(3)*m(3))+(l(3)*m(4))+(l(3)*m(5)))*(l(2)*sin(q(3))*q_d(2)) -((lc(4)*m(4))+(l(4)*m(5)))*(l(2)*sin(q(3)+q(4))*q_d(2))-((lc(3)*m(3))+(l(3)*m(4))+(l(3)*m(5)))*(l(2)*sin(q(3))*q_d(3)) - ((lc(4)*m(4))+(l(4)*m(5)))*(l(2)*sin(q(3)+q(4))*q_d(3))-((lc(4)*m(4))+(l(4)*m(5)))*((l(3)*sin(q(4)))+(l(2)*sin(q(3)+q(4)))*q_d(4));
V(2,4) = -((lc(4)*m(4))+(l(4)*m(5)))*((l(3)*sin(q(4)))+(l(2)*sin(q(3)+q(4))))*(q_d(3)+q_d(4)+q_d(2));
V(3,2) = ((lc(3)*m(3))+(l(3)*m(4))+(l(3)*m(5)))*(l(2)*sin(q(3))*q_d(2)) + ((lc(4)*m(4))+(l(4)*m(5)))*(l(2)*sin(q(3)+q(4))*q_d(2))-((lc(4)*m(4))+(l(4)*m(5)))*l(3)*sin(q(4))*q_d(4);
V(3,3) = -((lc(4)*m(4))+l(4)*m(5))*l(3)*sin(q(4))*q_d(4);
V(3,4) = -((lc(4)*m(4))+l(4)*m(5))*l(3)*sin(q(4))*(q_d(2)+q_d(3)+q_d(4));
V(4,2) = ((lc(4)*m(4))+l(4)*m(5))*((((l(2)*sin(q(3)+q(4)))+(l(3)*sin(q(4))))*q_d(2)) + (l(3)*sin(q(4))*q_d(3)));
V(4,3) =  ((lc(4)*m(4))+l(4)*m(5))*l(3)*sin(q(4))*(q_d(2)+q_d(3));

%%
gz= 9.8;
G = zeros(5,1);
%Populating gravitational force (G) matrix
G = [sum(m)*gz; 0; 0; 0; -m(5)*gz];

%%

F = zeros(5,1);
%Populating Friction (F) matrix
F = [(Fv(1)*q_d(1)); (Fv(2)*q_d(2)); (Fv(3)*q_d(3)); (Fv(4)*q_d(4)); (Fv(5)*q_d(5))];

end

== matlab function model1/Input Trajectory ==
  data: t input; y output
function y = fcn(t)

y = zeros(5,1);
y(1) = 0.5*t;
y(2) = 0.5*sin(2*t);
y(3) = - y(2);
y(4) = -0.5 + (0.5*cos(2*t));
y(5) = 0.375*t;

y = y(:);
end

== matlab function model1/Input Trajectory1 ==
  data: t input; y output
function y = fcn(t)

y = zeros(5,1);
y(1) = 0.5*t;
y(2) = 0.5*sin(2*t);
y(3) = - y(2);
y(4) = -0.5 + (0.5*cos(2*t));
y(5) = 0.375*t;

y = y(:);

end
